simulink model "verify_Storage_Type_0_mdl"  (R2018b)
settings: Solver=ode45  StartTime=0  StopTime=3*3600  MaxStep=600  RelTol=1e-3  EnableMultiTasking=on
undefined symbols (not defined in the file or in its folder): path_carnot
libraries: carnot x4, simulink x2
settings Model: Creator=drhf  LastModifiedBy=P41573
settings DataIOCC: SaveFormat=Array  SignalLoggingSaveFormat=ModelDataLogs
settings OptimizationCC: ExpressionDepthLimit=2147483647  LifeSpan=inf
settings DebuggingCC: UnderspecifiedInitializationDetection=Classic  MergeDetectMultiDrivingBlocksExec=none  SolverPrmCheckMsg=warning  FcnCallInpInsideContextMsg=warning  StateNameClashWarn=warning  SFUnexpectedBacktrackingDiag=warning  SFNoUnconditionalDefaultTransitionDiag=warning  SFExecutionAtInitializationDiag=none
settings HardwareCC: ProdBitPerPointer=32  ProdBitPerSizeT=32  ProdBitPerPtrDiffT=32  ProdLargestAtomicFloat=None  ProdIntDivRoundTo=Undefined  ProdEndianess=Unspecified  ProdWordSize=32  ProdHWDeviceType=32-bit Generic
settings ModelReferenceCC: PropagateSignalLabelsOutOfModel=off
settings SFSimCC: SimUseLocalCustomCode=off
settings RTWCC: RTWUseLocalCustomCode=off
settings CodeAppCC: StateflowObjectComments=on
settings GRTTargetCC: TargetLangStandard=C89/C90 (ANSI)  GeneratePreprocessorConditionals=Disable all  CombineOutputUpdateFcns=off  GRTInterface=on
settings ConfigComp: CovMetricSettings=dw  CovHtmlReporting=on  CovSaveCumulativeToWorkspaceVar=on  CovSaveSingleToWorkspaceVar=on  CovExternalEMLEnable=off

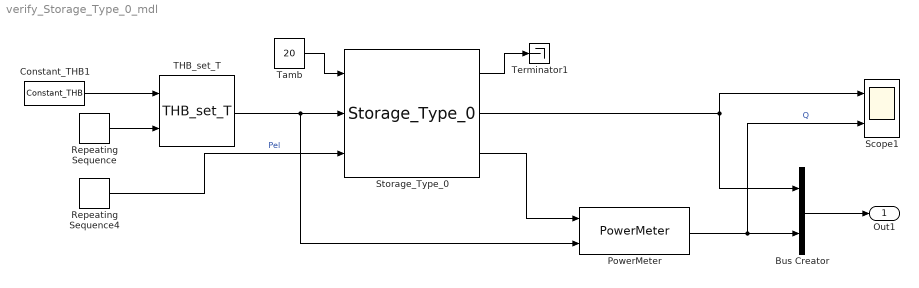
== system verify_Storage_Type_0_mdl ==
  Bus Creator : BusCreator  Inputs=2
  Constant_THB1 : carnot/Source/Simple/Constant_THB  t=30  mdot=900/3600  p=1e5  mID=No Pressure Drop  fluid=Water (Constant 20°C)  mix=0  mix2=0  mix3=0  dia=0.02  hgt=0
  PowerMeter : carnot/Control/PowerMeter
  Repeating Sequence : simulink/Sources/Repeating Sequence  rep_seq_t=[0 1.5*3600 1.5*3600+1 3*3600]  rep_seq_y=[20 20 30 30]
  Repeating Sequence4 : simulink/Sources/Repeating Sequence  rep_seq_t=[ 0 7200 7200+eps(7200) 10800 10800+eps(10800) 14600]  rep_seq_y="[ 0   0     3e3                  3e3     0                    0]"
  Scope1 : Scope  NumInputPorts=2
  Storage_Type_0 : carnot/Storage/Thermal/Storage_Type_0  t0=20  hgt=1.5279  stgtype=0  mpts=[1 2 3 4 5 6 7 8 9 10]  tini=[20 20 20 20 20 20 20 20 20 20]  PathName=fullfile(path_carnot('libsl'),'Storage','Thermal','Storage_Type_0','parameter_set')  FileName='StorageTyp0_300_L.mat'  userPath=off  userParam=off  uwall=1  ubot=1  utop=1  axcond=1  volume=0.3  dia=0.5  standing=standing cylinder  nodes=10  mpoints=10  Tsensor=0.5  pipe1inlet=1  pipe1outlet=0  pipe1dia=0.03  heater1start=0.2  heater1end=0.25
  THB_set_T : carnot/Source/Simple/THB_set_T
  Tamb : Constant  Value=20
  Terminator1 : Terminator
  Out1 : Outport
  wires:
  THB_set_T/1 -> Storage_Type_0/2, PowerMeter/2
  Bus Creator/1 -> Out1/1
  Storage_Type_0/1 -> Terminator1/1
  PowerMeter/1 -> Bus Creator/2, Scope1/2  "Q"
  Tamb/1 -> Storage_Type_0/1
  Storage_Type_0/3 -> PowerMeter/1
  Storage_Type_0/2 -> Scope1/1, Bus Creator/1
  Constant_THB1/1 -> THB_set_T/1
  Repeating Sequence/1 -> THB_set_T/2
  Repeating Sequence4/1 -> Storage_Type_0/3  "Pel"
